simulink model "test"  (R2016b)
settings: Solver=VariableStepAuto  StartTime=0.0  StopTime=inf  RelTol=1e-3
settings Model: Creator=gaoweijin  LastModifiedBy=gaoweijin

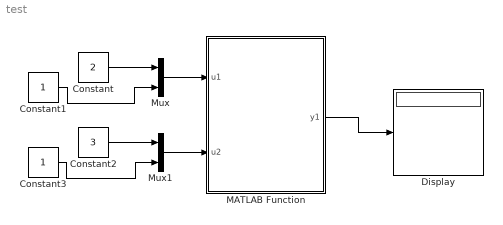
== system test ==
  Constant : Constant  Value=2
  Constant1 : Constant
  Constant2 : Constant  Value=3
  Constant3 : Constant
  Display : Display
  MATLAB Function : MATLAB Function  TreatAsAtomicUnit=on
  Mux : Mux  Inputs=2
  Mux1 : Mux  Inputs=2
  wires:
  Constant/1 -> Mux/1
  Constant1/1 -> Mux/2
  Constant2/1 -> Mux1/1
  Constant3/1 -> Mux1/2
  Mux1/1 -> MATLAB Function/2(u2)
  Mux/1 -> MATLAB Function/1(u1)
  MATLAB Function/1(y1) -> Display/1

== matlab function test/MATLAB Function ==
  data: u1 input; y1 output; u2 input
function y1 = fcn(u1,u2)
temp = zeros(2,1);
temp(1) = u1(1) + u1(2);
temp(2) = u2(1) + u2(2);
y1 = temp;
